simulink model "Filtro_teste_potencia_constante"  (R2014b)
settings: Solver=ode45  StartTime=0.0  StopTime=0.05  MaxStep=1e-6  RelTol=1e-3
undefined symbols (not defined in the file or in its folder): wc
libraries: powerlib x21, powerlib_meascontrol x3
settings Model: Creator=JPSOLIV  LastModifiedBy=JPSOLIV

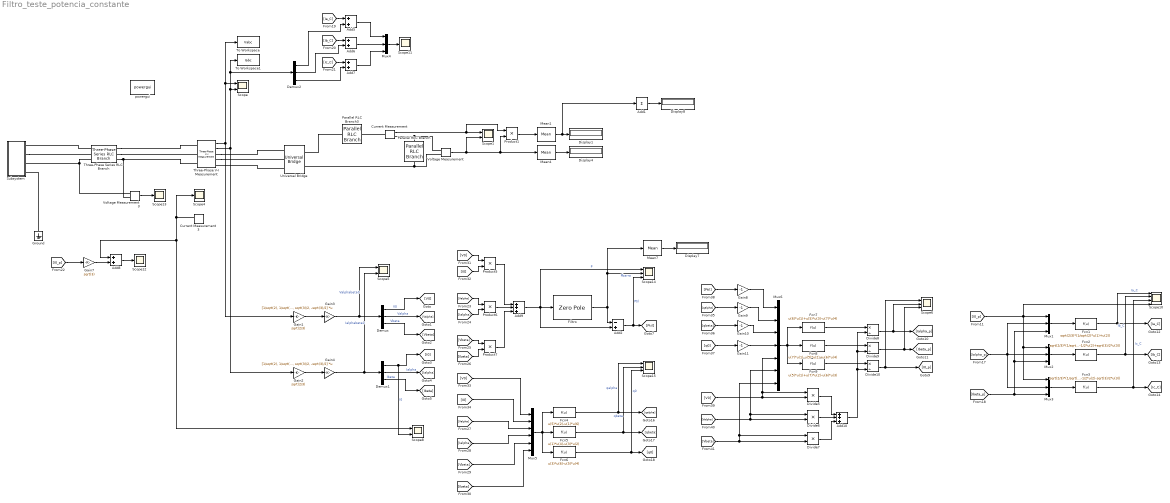
== system Filtro_teste_potencia_constante ==
  Add1 : Sum  Inputs=+
  Add10 : Sum  Inputs=+++
  Add2 : Sum  Inputs=-+
  Add{5..8} (4 alike) : Sum
  Add9 : Sum  Inputs=+++
  Current Measurement : powerlib/Measurements/Current Measurement  PhasorSimulation=off  OutputType=Complex  PSBequivalent=0
  Current Measurement3 : powerlib/Measurements/Current Measurement  PhasorSimulation=off  OutputType=Complex  PSBequivalent=0
  Demux : Demux  Outputs=3
  Demux1 : Demux  Outputs=3
  Demux2 : Demux  Outputs=3
  Display{1,4,7..8} (4 alike) : Display
  Divide10 : Product  Inputs=*/
  Divide5 : Product  Inputs=**
  Divide6 : Product  Inputs=**
  Divide7 : Product  Inputs=**
  Divide8 : Product  Inputs=*/
  Divide9 : Product  Inputs=*/
  Fcn1 : Fcn  Expr=sqrt(2/3)*(1/sqrt(2)*u(1)+u(2))
  Fcn2 : Fcn  Expr=sqrt(2/3)*(1/sqrt(2)*u(1)-1/2*u(2)+sqrt(3)/2*u(3))
  Fcn3 : Fcn  Expr=sqrt(2/3)*(1/sqrt(2)*u(1)-1/2*u(2)-sqrt(3)/2*u(3))
  Fcn4 : Fcn  Expr=u(5)*u(2)-u(1)*u(6)
  Fcn5 : Fcn  Expr=u(1)*u(4)-u(3)*u(2)
  Fcn6 : Fcn  Expr=u(3)*u(6)-u(5)*u(4)
  Fcn7 : Fcn  Expr=u(6)*u(1)+u(5)*u(3)-u(7)*u(4)
  Fcn8 : Fcn  Expr=u(7)*u(1)-u(5)*u(2)+u(6)*u(4)
  Fcn9 : Fcn  Expr=u(5)*u(1)+u(7)*u(2)-u(6)*u(3)
  Filtro : ZeroPole  Zeros=[]  Poles=[-wc -wc -wc -wc]  Gain=[wc^4]
  Gain1 : Gain  Gain=sqrt(2/3)
  Gain{8..11} (4 alike) : Gain  Gain=-1
  Gain2 : Gain  Gain=sqrt(2/3)
  Gain3 : Gain  Gain=[1/sqrt(2), 1/sqrt(2), 1/sqrt(2); 1, -1/2, -1/2; 0, sqrt(3)/2, -sqrt(3)/2]  Multiplication=Matrix(K*u)
  Gain4 : Gain  Gain=[1/sqrt(2), 1/sqrt(2), 1/sqrt(2); 1, -1/2, -1/2; 0, sqrt(3)/2, -sqrt(3)/2]  Multiplication=Matrix(K*u)
  Gain7 : Gain  Gain=sqrt(3)
  Ground : powerlib/Elements/Ground  LConnTagsString=a
  Mean1 : powerlib_meascontrol/Measurements/Mean  Freq=400  Vinit=0  Ts=0
  Mean4 : powerlib_meascontrol/Measurements/Mean  Freq=400  Vinit=0  Ts=0
  Mean7 : powerlib_meascontrol/Measurements/Mean  Freq=400  Vinit=0  Ts=0
  Mux{1..4} (4 alike) : Mux  Inputs=3
  Mux5 : Mux  Inputs=6
  Mux6 : Mux  Inputs=7
  Parallel RLC Branch : powerlib/Elements/Parallel RLC Branch  LConnTagsString=a  RConnTagsString=__new0  BranchType=RC  Resistance=50  Inductance=1e-3  SetiL0=off  InitialCurrent=0  Capacitance=30e-6  Setx0=off  InitialVoltage=0  Measurements=None
  Parallel RLC Branch3 : powerlib/Elements/Parallel RLC Branch  LConnTagsString=a  RConnTagsString=__new0  BranchType=L  Resistance=1  Inductance=10e-3  SetiL0=off  InitialCurrent=0  Capacitance=30e-6  Setx0=off  InitialVoltage=0  Measurements=None
  Product{1,5..7} (4 alike) : Product
  Scope{,1,5,8} (4 alike) : Scope  NumInputPorts=2
      Scope settings: YMin=-6~-0.8  YMax=6~0.8
      Scope1 settings: YMin=-0.00169333~0  YMax=20~200
      Scope5 settings: YMin=-600~-200  YMax=400~200  SaveName=ScopeData5
      Scope8 settings: YMin=-600~-200  YMax=400~200  SaveName=ScopeData8
  Scope10 : Scope  NumInputPorts=4
      settings: YMin=-8~-22.5~-10~-15  YMax=8~22.5~10~15  SaveName=ScopeData10
  Scope{4,11..13} (4 alike) : Scope
      Scope11 settings: YMin=-9  YMax=9  SaveName=ScopeData11
      Scope12 settings: YMin=-1.5e-09  YMax=1.5e-09  SaveName=ScopeData12
      Scope13 settings: YMin=-25  YMax=27.5  SaveName=ScopeData13
      Scope4 settings: YMin=-25  YMax=27.5  SaveName=ScopeData4
  Scope14 : Scope  NumInputPorts=3
      settings: YMin=0~0~-1500  YMax=3000~2000~1750  SaveName=ScopeData15
  Scope15 : Scope  NumInputPorts=3
      settings: YMin=0~0~-5000  YMax=105000~5000~105000  SaveName=ScopeData16
  Scope6 : Scope  NumInputPorts=3
      settings: YMin=-15~-15~-20  YMax=15~15~20  SaveName=ScopeData6
  Subsystem : Subsystem  mask{Vp=115*sqrt(2), Vn=0, phin=0, Vz=0, phi0=0, f=400}
      mask prompts: Vp "Tensão Sequência Positiva"; Vn "Tensão Sequência Negativa"; phin "Defasagem Sequência Negativa"; Vz "Tensão Sequência Zero"; phi0 "Defasagem Sequência Zero"; f "Frequência"
  Three-Phase Series RLC Branch : powerlib/Elements/Three-Phase Series RLC Branch  LConnTagsString=A|B|C  RConnTagsString=A|B|C  BranchType=RL  Resistance=eps  Inductance=eps  Capacitance=1e-6  Measurements=None
  Three-Phase V-I Measurement : powerlib/Measurements/Three-Phase V-I Measurement  VoltageMeasurement=phase-to-ground  SetLabelV=off  LabelV=Vabc  Vpu=off  VpuLL=off  CurrentMeasurement=yes  SetLabelI=off  LabelI=Iabc  Ipu=off  Pbase=100e6  Vbase=500e3  OutputType=Complex  PhasorSimulation=off  PSBequivalent=0
  To Workspace : ToWorkspace  VariableName=Vabc  SaveFormat=Structure With Time  SampleTime=-1
  To Workspace1 : ToWorkspace  VariableName=Iabc  SaveFormat=Structure With Time  SampleTime=-1
  Universal Bridge : powerlib/Power Electronics/Universal Bridge  Arms=3  SnubberResistance=1e5  SnubberCapacitance=inf  Device=Diodes  Ron=1e-3  Lon=0  ForwardVoltages="[  0  0  ]"  ForwardVoltage=0  GTOparameters=[ 10e-6 , 20e-6 ]  IGBTparameters=[ 1e-6 , 2e-6 ]  Measurements=None  Measurements_2=None  converterType=Rectifier
  Voltage Measurement : powerlib/Measurements/Voltage Measurement  PhasorSimulation=off  OutputType=Complex  PSBequivalent=0
  Voltage Measurement3 : powerlib/Measurements/Voltage Measurement  PhasorSimulation=off  OutputType=Complex  PSBequivalent=0
  powergui : powerlib/powergui  Priority=1  SimulationMode=Discrete  SolverType=Tustin  SampleTime=5e-7  frequency=60  SPID=off  DisableSnubberDevices=off  DisableRonSwitches=off  DisableVfSwitches=off  SwTol=0  DisplayEquations=off  Interpol=off  methode=off  Ts=100  frequencyindice=0  Pbase=100e6  ErrMax=1e-4  Iterations=50  UnitsV=kV  UnitsW=MW  FunctionMessages=off  echomessages=off  HookPort=off  EnableUseOfTLC=off  x0status=blocks  RestoreLinks=warning  ResistiveCurrentMeasurement=off  Frange=[0:2:500]  Ylog=off  Xlog=on  ShowGrid=off  save=off  variable=ZData  structure=0  ZoomFFT=off  StartTime=0.0  cycles=1  DisplayStyle=1  fundamental=60  FreqAxis=off  MaxFrequency=1000  frequencyindicesteady=1  RmsSteady=1  display=off
  wires:
  Three-Phase V-I Measurement/1 -> To Workspace/1, Scope/1, Gain1/1
  Three-Phase V-I Measurement/2 -> Gain2/1, Demux2/1, To Workspace1/1, Scope/2
  Gain1/1 -> Gain3/1
  Gain2/1 -> Gain4/1
  Gain3/1 -> Demux/1, Scope5/1  "Valphabeta0"
  Gain4/1 -> Scope5/2, Demux1/1  "Ialphabeta0"
  Demux/1 -> [V0]  "V0"
  Demux/2 -> [Valpha]  "Valpha"
  Demux1/2 -> [Ialpha]  "Ialpha"
  Demux/3 -> [Vbeta]  "Vbeta"
  Demux1/3 -> [Ibeta]  "Ibeta"
  Demux1/1 -> Scope8/2, [I0]  "I0"
  Mux1/1 -> Fcn1/1
  [I0_p] -> Scope10/4, Mux2/1, Mux3/1, Mux1/1
  [Ialpha_p] -> Mux3/2, Mux2/2, Mux1/2
  [Ibeta_p] -> Mux3/3, Mux1/3, Mux2/3
  Fcn1/1 -> [Ia_C], Scope10/1  "Ia_C"
  Mux2/1 -> Fcn2/1
  Fcn2/1 -> [Ib_C], Scope10/2  "Ib_C"
  Mux3/1 -> Fcn3/1
  Fcn3/1 -> [Ic_C], Scope10/3  "Ic_C"
  [Ia_C] -> Add5/1
  [Ib_C] -> Add6/1
  [Ic_C] -> Add7/1
  Demux2/1 -> Add5/2
  Demux2/2 -> Add6/2
  Demux2/3 -> Add7/2
  Add6/1 -> Mux4/2
  Mux4/1 -> Scope11/1
  [I0_p] -> Gain7/1
  Current Measurement3/1 -> Scope4/1, Scope8/1, Add8/1
  Add8/1 -> Scope12/1
  Gain7/1 -> Add8/2
  Add7/1 -> Mux4/3
  Add5/1 -> Mux4/1
  Voltage Measurement3/1 -> Scope13/1
  [V0] -> Product5/1
  [I0] -> Product5/2
  [Valpha] -> Product6/1
  [Ialpha] -> Product6/2
  [Vbeta] -> Product7/1
  [Ibeta] -> Product7/2
  Product6/1 -> Add9/2
  Product5/1 -> Add9/1
  Product7/1 -> Add9/3
  Mux5/1 -> Fcn4/1, Fcn6/1, Fcn5/1
  [V0] -> Mux5/1
  [I0] -> Mux5/2
  [Valpha] -> Mux5/3
  [Ialpha] -> Mux5/4
  [Vbeta] -> Mux5/5
  [Ibeta] -> Mux5/6
  Fcn4/1 -> [qalpha], Scope15/1  "qalpha"
  Fcn5/1 -> [qbeta], Scope15/2  "qbeta"
  Fcn6/1 -> [q0], Scope15/3  "q0"
  Add9/1 -> Add2/2, Filtro/1, Scope14/1  "P"
  Filtro/1 -> Add2/1, Mean7/1, Scope14/2  "Pbarra"
  Add2/1 -> Scope14/3, [Ptil]  "Ptil"
  [Ptil] -> Gain8/1
  [qalpha] -> Gain9/1
  [qbeta] -> Gain10/1
  [q0] -> Gain11/1
  Gain8/1 -> Mux6/1
  Gain9/1 -> Mux6/2
  Gain10/1 -> Mux6/3
  Gain11/1 -> Mux6/4
  [V0] -> Mux6/5, Divide5/1, Divide5/2
  [Valpha] -> Mux6/6, Divide6/1, Divide6/2
  [Vbeta] -> Mux6/7, Divide7/1, Divide7/2
  Divide5/1 -> Add10/1
  Divide6/1 -> Add10/2
  Divide7/1 -> Add10/3
  Mux6/1 -> Fcn7/1, Fcn9/1, Fcn8/1
  Fcn7/1 -> Divide8/1
  Fcn8/1 -> Divide9/1
  Fcn9/1 -> Divide10/1
  Add10/1 -> Divide10/2, Divide9/2, Divide8/2
  Divide9/1 -> Scope6/3, [Ibeta_p]
  Divide10/1 -> Scope6/1, [I0_p]
  Divide8/1 -> Scope6/2, [Ialpha_p]
  Current Measurement/1 -> Product1/1, Scope1/1
  Voltage Measurement/1 -> Scope1/2, Product1/2, Mean4/1
  Product1/1 -> Mean1/1
  Mean1/1 -> Add1/1, Display1/1
  Mean4/1 -> Display4/1
  Mean7/1 -> Display7/1
  Add1/1 -> Display8/1
  connections:
  Parallel RLC Branch/RConn1 -- Universal Bridge/RConn2 -- Voltage Measurement/LConn2
  Three-Phase V-I Measurement/RConn1 -- Universal Bridge/LConn1
  Current Measurement/RConn1 -- Voltage Measurement/LConn1 -- Parallel RLC Branch/LConn1
  Parallel RLC Branch3/RConn1 -- Universal Bridge/RConn1
  Three-Phase Series RLC Branch/RConn2 -- Three-Phase V-I Measurement/LConn2
  Three-Phase Series RLC Branch/RConn1 -- Three-Phase V-I Measurement/LConn1
  Three-Phase Series RLC Branch/RConn3 -- Voltage Measurement3/LConn2 -- Three-Phase V-I Measurement/LConn3
  Current Measurement/LConn1 -- Parallel RLC Branch3/LConn1
  Ground/LConn1 -- Subsystem/RConn4
  Voltage Measurement3/LConn1 -- Three-Phase Series RLC Branch/LConn3 -- Subsystem/RConn3
  Subsystem/RConn2 -- Three-Phase Series RLC Branch/LConn2
  Three-Phase Series RLC Branch/LConn1 -- Subsystem/RConn1
  Three-Phase V-I Measurement/RConn2 -- Universal Bridge/LConn2
  Universal Bridge/LConn3 -- Three-Phase V-I Measurement/RConn3

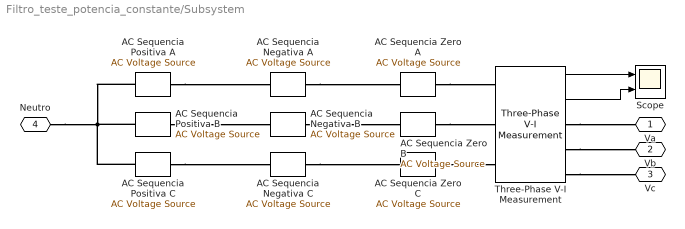
== system Filtro_teste_potencia_constante/Subsystem ==
  AC Sequencia Negativa A : powerlib/Electrical Sources/AC Voltage Source  Amplitude=Vn  Phase=0+phin  Frequency=f  SampleTime=0  Measurements=None
  AC Sequencia Negativa B : powerlib/Electrical Sources/AC Voltage Source  Amplitude=Vn  Phase=120+phin  Frequency=f  SampleTime=0  Measurements=None
  AC Sequencia Negativa C : powerlib/Electrical Sources/AC Voltage Source  Amplitude=Vn  Phase=-120+phin  Frequency=f  SampleTime=0  Measurements=None
  AC Sequencia Positiva A : powerlib/Electrical Sources/AC Voltage Source  Amplitude=Vp  Phase=0  Frequency=f  SampleTime=0  Measurements=None
  AC Sequencia Positiva B : powerlib/Electrical Sources/AC Voltage Source  Amplitude=Vp  Phase=-120  Frequency=f  SampleTime=0  Measurements=None
  AC Sequencia Positiva C : powerlib/Electrical Sources/AC Voltage Source  Amplitude=Vp  Phase=+120  Frequency=f  SampleTime=0  Measurements=None
  AC Sequencia Zero A : powerlib/Electrical Sources/AC Voltage Source  Amplitude=Vz  Phase=0+phi0  Frequency=f  SampleTime=0  Measurements=None
  AC Sequencia Zero B : powerlib/Electrical Sources/AC Voltage Source  Amplitude=Vz  Phase=0+phi0  Frequency=f  SampleTime=0  Measurements=None
  AC Sequencia Zero C : powerlib/Electrical Sources/AC Voltage Source  Amplitude=Vz  Phase=0+phi0  Frequency=f  SampleTime=0  Measurements=None
  Scope : Scope  NumInputPorts=2
      settings: YMin=-6~-0.8  YMax=6~0.8  SaveName=ScopeData14
  Three-Phase V-I Measurement : powerlib/Measurements/Three-Phase V-I Measurement  VoltageMeasurement=phase-to-ground  SetLabelV=off  LabelV=Vabc  Vpu=off  VpuLL=off  CurrentMeasurement=yes  SetLabelI=off  LabelI=Iabc  Ipu=off  Pbase=100e6  Vbase=500e3  OutputType=Complex  PhasorSimulation=off  PSBequivalent=0
  Va : PMIOPort  Port=1  Side=Right
  Vb : PMIOPort  Port=2  Side=Right
  Vc : PMIOPort  Port=3  Side=Right
  Neutro : PMIOPort  Port=4  Side=Right
  wires:
  Three-Phase V-I Measurement/1 -> Scope/1
  Three-Phase V-I Measurement/2 -> Scope/2
  connections:
  AC Sequencia Positiva A/LConn1 -- Neutro/RConn1 -- AC Sequencia Positiva C/LConn1 -- AC Sequencia Positiva B/LConn1
  AC Sequencia Positiva C/RConn1 -- AC Sequencia Negativa C/LConn1
  AC Sequencia Positiva B/RConn1 -- AC Sequencia Negativa B/LConn1
  AC Sequencia Positiva A/RConn1 -- AC Sequencia Negativa A/LConn1
  AC Sequencia Negativa A/RConn1 -- AC Sequencia Zero A/LConn1
  AC Sequencia Negativa B/RConn1 -- AC Sequencia Zero B/LConn1
  AC Sequencia Negativa C/RConn1 -- AC Sequencia Zero C/LConn1
  AC Sequencia Zero A/RConn1 -- Three-Phase V-I Measurement/LConn1
  AC Sequencia Zero B/RConn1 -- Three-Phase V-I Measurement/LConn2
  AC Sequencia Zero C/RConn1 -- Three-Phase V-I Measurement/LConn3
  Three-Phase V-I Measurement/RConn1 -- Va/RConn1
  Three-Phase V-I Measurement/RConn2 -- Vb/RConn1
  Three-Phase V-I Measurement/RConn3 -- Vc/RConn1
